simulink model "model_trapezoidal_gust_test"  (R2020b)
settings: configuration reference "Configuration" (kept outside this file)
settings Model: NumberOfSteps=10  Creator=dogukan  LastModifiedBy=dogukan
settings ConfigSetRef: SourceName=Configuration  SourceLocation=Base Workspace

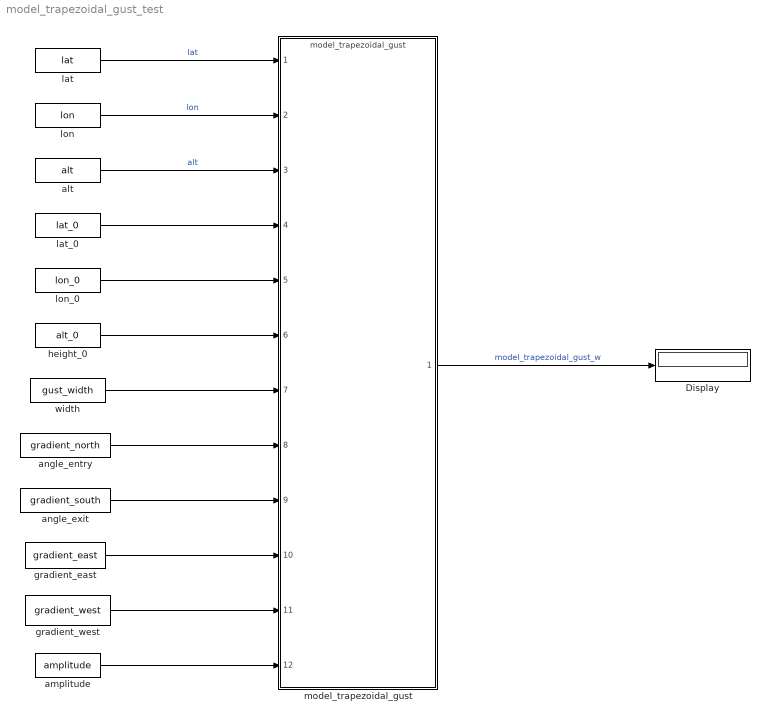
== system model_trapezoidal_gust_test ==
  Display : Display
  alt : FromWorkspace  VariableName=alt
  amplitude : FromWorkspace  VariableName=amplitude
  angle_entry : FromWorkspace  VariableName=gradient_north
  angle_exit : FromWorkspace  VariableName=gradient_south
  gradient_east : FromWorkspace  VariableName=gradient_east
  gradient_west : FromWorkspace  VariableName=gradient_west
  height_0 : FromWorkspace  VariableName=alt_0
  lat : FromWorkspace  VariableName=lat
  lat_0 : FromWorkspace  VariableName=lat_0
  lon : FromWorkspace  VariableName=lon
  lon_0 : FromWorkspace  VariableName=lon_0
  model_trapezoidal_gust : ModelReference  ModelNameDialog=model_trapezoidal_gust.slx  SimulationMode=Normal  ModelReferenceVersion=1.145
  width : FromWorkspace  VariableName=gust_width
  wires:
  lat/1 -> model_trapezoidal_gust/1  "lat"
  lon/1 -> model_trapezoidal_gust/2  "lon"
  alt/1 -> model_trapezoidal_gust/3  "alt"
  height_0/1 -> model_trapezoidal_gust/6
  lon_0/1 -> model_trapezoidal_gust/5
  lat_0/1 -> model_trapezoidal_gust/4
  model_trapezoidal_gust/1 -> Display/1  "model_trapezoidal_gust_w"
  width/1 -> model_trapezoidal_gust/7
  angle_entry/1 -> model_trapezoidal_gust/8
  angle_exit/1 -> model_trapezoidal_gust/9
  gradient_west/1 -> model_trapezoidal_gust/11
  gradient_east/1 -> model_trapezoidal_gust/10
  amplitude/1 -> model_trapezoidal_gust/12
